simulink model "Vehicle_Model_Controller_Dec26"  (R2020b)
settings: Solver=VariableStepAuto  StartTime=0.0  StopTime=30  FixedStep=0.015  MaxStep=0.1  RelTol=1e-3
model workspace (MAT data in the model file):
  Kp = 10
  understeer_gradient = 0.05
undefined symbols (not defined in the file): BWL, BWR, FWL, FWR
libraries: fl_lib x32, nesl_utility x24, sdl_lib x8, pid_lib x1, vehdynlibsteering x1, autolibshared x1, autolibdatasheetbattery x1
(part 2 of 2)

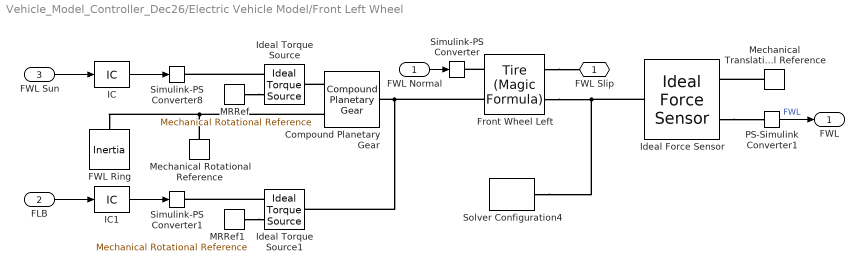
== system Vehicle_Model_Controller_Dec26/Electric Vehicle Model/Front Left Wheel ==
  FWL Normal : Inport
  FLB : Inport  Port=2
  FWL Sun : Inport  Port=3
  Compound Planetary Gear : sdl_lib/Gears/Compound Planetary Gear  rp_ratio=84/23  ps_ratio=37/24  friction_model=sdl.enum.gear_friction.none  mu_visc=[0, 0] N*m/(rad/s)  efficiency=[.96, .98]  temperature_TLU=[280, 300, 320] K  efficiency_sp_TLU=[.95, .9, .85]  efficiency_rp_TLU=[.95, .9, .85]  pwr_thr=[.001, .001] W  thermal_mass=50 J/K  T_init=300 K  model_inertia=simscape.enum.onoff.off  planet_inertia=0.001 kg*m^2
      settings: SourceProductBaseCode=LD  InternalSimscapePortConfiguration="{\"Bottom\":[],\"Left\":[{\"id\":\"C\",\"label\":\"C\",\"type\":\"foundation.mechanical.rotational.rotational\"}],\"Right\":[{\"id\":\"R\",\"label\":\"R\",\"type\":\"foundation.mechanical.rotational.rotational\"},{\"id\":\"S\",\"label\":\"S\",\"type\":\"foundation.mechanical.rotational.rotational\"}],\"Top\":[]}"
  FWL Ring : fl_lib/Mechanical/Rotational Elements/Inertia  inertia=0.1 kg*m^2  num_ports=foundation.enum.numPorts2.one  w_specify=off  w_priority=High  w=0 rad/s  w_nominal_specify=off  w_nominal_unit=rad/s  w_nominal_value=1  t_specify=off  t_priority=None  t=0 N*m  t_nominal_specify=off  t_nominal_unit=N*m  t_nominal_value=1
  Front Wheel Left : sdl_lib/Tires & Vehicles/Tire (Magic Formula)  parameterization=sdl.enum.magic_tire_model.constant  F_z1=3000 N  F_x1=3500 N  kappa1=10  B_m=10  C_m=1.9  D_m=1.5  E_m=0.97  fz0=4000 N  p_Cx=1.685  p_Dx=[1.21, -.037]  p_Ex=[.344, .095, -.02, 0]  p_Kx=[21.51, -.163, .245]  p_Hx=[-.002, .002]  p_Vx=[0, 0]  v_tr_thr=0.1 m/s  r_e=0.22 m  model_compliance=1  stiffness=2e5 N/m  damping=1000 N/(m/s)  model_inertia=1  inertia=0.03 kg*m^2  initial_velocity=0 rad/s  model_resistance=1  resistance_model=1  coeff=0.015  p_tire=82.74e3 Pa  alpha=-0.003  beta=0.97  coeff_a=84e-4  coeff_b=6.2e-4 s/m  coeff_c=1.6e-4 s^2/m^2  v_thr=0.01 m/s
  IC : InitialCondition  Value=0
  IC1 : InitialCondition  Value=0
  Ideal Force Sensor : fl_lib/Mechanical/Mechanical Sensors/Ideal Force Sensor
  Ideal Torque Source : fl_lib/Mechanical/Mechanical Sources/Ideal Torque Source
      settings: SourceProductName=Foundation Library
  Ideal Torque Source1 : fl_lib/Mechanical/Mechanical Sources/Ideal Torque Source
      settings: SourceProductName=Foundation Library
  MRRef : fl_lib/Mechanical/Rotational Elements/Mechanical Rotational Reference
      settings: SourceProductName=Foundation Library
  MRRef1 : fl_lib/Mechanical/Rotational Elements/Mechanical Rotational Reference
      settings: SourceProductName=Foundation Library
  Mechanical Rotational Reference : fl_lib/Mechanical/Rotational Elements/Mechanical Rotational Reference
  Mechanical Translational Reference : fl_lib/Mechanical/Translational Elements/Mechanical Translational Reference
  PS-Simulink Converter1 : nesl_utility/PS-Simulink Converter  PhysicalDomain=network_engine_domain  SubClassName=ps_output  LeftPortType=input  RightPortType=output  PseudoPeriodic=off  Frequencies=[]  Unit=inherit  AffineConversion=off
      settings: SourceProductBaseCode=PW,SS
  Simulink-PS Converter : nesl_utility/Simulink-PS Converter  PhysicalDomain=network_engine_domain  SubClassName=ps_input  LeftPortType=input  RightPortType=output  PseudoPeriodic=off  Frequencies=[]  NoiseDistribution=none  NoiseParameters=[]  Unit=N  AffineConversion=off  FilteringAndDerivatives=zero  SimscapeFilterOrder=1  InputFilterTimeConstant=0.001  UdotUserProvided=0
      settings: SourceProductBaseCode=PW,SS
  Simulink-PS Converter1 : nesl_utility/Simulink-PS Converter  PhysicalDomain=network_engine_domain  SubClassName=ps_input  LeftPortType=input  RightPortType=output  PseudoPeriodic=off  Frequencies=[]  NoiseDistribution=none  NoiseParameters=[]  Unit=N*m  AffineConversion=off  FilteringAndDerivatives=zero  SimscapeFilterOrder=1  InputFilterTimeConstant=0.001  UdotUserProvided=0
      settings: SourceProductBaseCode=PW,SS
  Simulink-PS Converter8 : nesl_utility/Simulink-PS Converter  PhysicalDomain=network_engine_domain  SubClassName=ps_input  LeftPortType=input  RightPortType=output  PseudoPeriodic=off  Frequencies=[]  NoiseDistribution=none  NoiseParameters=[]  Unit=N*m  AffineConversion=off  FilteringAndDerivatives=zero  SimscapeFilterOrder=1  InputFilterTimeConstant=0.001  UdotUserProvided=0
      settings: SourceProductBaseCode=PW,SS
  Solver Configuration4 : nesl_utility/Solver Configuration  PhysicalDomain=network_engine_domain  SubClassName=solver  LeftPortType=input  RightPortType=generic  Tones=[]  Harmonics=[]  SimulateNoise=off  Profile=off  UseLocalSampling=off  EnableSwitchedLinearOptims=on  FrequencyDomain=off  UseCCode=off  RelTol=0.001  AbsTol=1e-06  MinStep=1e-09  ToWorkspace=off  RevertToSquareIcSolve=off  NumHomotopyIterations=100  PhasorMode=off  PhasorModeNumHarmonics=1  DoDC=off  ResidualTolerance=1e-09  UseLocalSolver=off  LocalSolverChoice=NE_BACKWARD_EULER_ADVANCER  LocalSolverSampleTime=0.001  DoFixedCost=on  MaxNonlinIter=200  MaxModeIter=20  ComputeImpulses=off  ImpulseIterations=20  LinearAlgebra=auto  EquationFormulation=NE_TIME_EF  DelaysMemoryBudget=1024  AutomaticFiltering=on  FilteringTimeConstant=0.001  PartitionStorageMethod=AS_NEEDED  PartitionMemoryBudget=1024  PartitionMethod=ROBUST
      settings: SourceProductBaseCode=PW,SS
  FWL Slip : PMIOPort  Side=Left
  FWL : Outport
  wires:
  PS-Simulink Converter1/1 -> FWL/1  "FWL"
  FWL Normal/1 -> Simulink-PS Converter/1
  IC/1 -> Simulink-PS Converter8/1
  FWL Sun/1 -> IC/1
  IC1/1 -> Simulink-PS Converter1/1
  FLB/1 -> IC1/1
  connections:
  Front Wheel Left/RConn1 -- FWL Slip/RConn1
  Ideal Force Sensor/RConn2 -- PS-Simulink Converter1/LConn1
  Ideal Force Sensor/LConn1 -- Front Wheel Left/RConn2 -- Solver Configuration4/RConn1
  Front Wheel Left/LConn1 -- Simulink-PS Converter/RConn1
  Mechanical Translational Reference/LConn1 -- Ideal Force Sensor/RConn1
  Mechanical Rotational Reference/LConn1 -- FWL Ring/LConn1 -- Compound Planetary Gear/RConn1
  Ideal Torque Source/RConn1 -- Simulink-PS Converter8/RConn1
  Compound Planetary Gear/RConn2 -- Ideal Torque Source/LConn1
  MRRef/LConn1 -- Ideal Torque Source/RConn2
  Ideal Torque Source1/RConn1 -- Simulink-PS Converter1/RConn1
  MRRef1/LConn1 -- Ideal Torque Source1/RConn2
  Front Wheel Left/LConn2 -- Ideal Torque Source1/LConn1 -- Compound Planetary Gear/LConn1

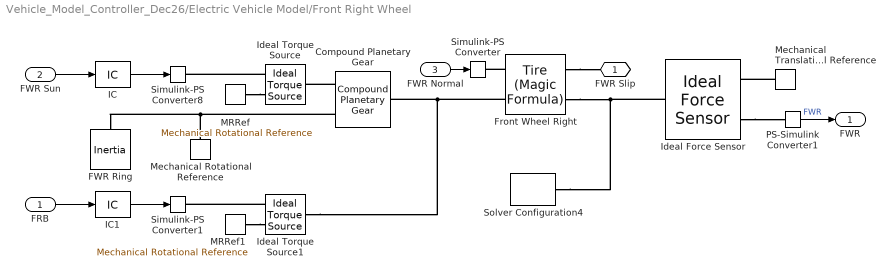
== system Vehicle_Model_Controller_Dec26/Electric Vehicle Model/Front Right Wheel ==
  FRB : Inport
  FWR Sun : Inport  Port=2
  FWR Normal : Inport  Port=3
  Compound Planetary Gear : sdl_lib/Gears/Compound Planetary Gear  rp_ratio=84/23  ps_ratio=37/24  friction_model=sdl.enum.gear_friction.none  mu_visc=[0, 0] N*m/(rad/s)  efficiency=[.96, .98]  temperature_TLU=[280, 300, 320] K  efficiency_sp_TLU=[.95, .9, .85]  efficiency_rp_TLU=[.95, .9, .85]  pwr_thr=[.001, .001] W  thermal_mass=50 J/K  T_init=300 K  model_inertia=simscape.enum.onoff.off  planet_inertia=0.001 kg*m^2
      settings: SourceProductBaseCode=LD  InternalSimscapePortConfiguration="{\"Bottom\":[],\"Left\":[{\"id\":\"C\",\"label\":\"C\",\"type\":\"foundation.mechanical.rotational.rotational\"}],\"Right\":[{\"id\":\"R\",\"label\":\"R\",\"type\":\"foundation.mechanical.rotational.rotational\"},{\"id\":\"S\",\"label\":\"S\",\"type\":\"foundation.mechanical.rotational.rotational\"}],\"Top\":[]}"
  FWR Ring : fl_lib/Mechanical/Rotational Elements/Inertia  inertia=0.1 kg*m^2  num_ports=foundation.enum.numPorts2.one  w_specify=off  w_priority=High  w=0 rad/s  w_nominal_specify=off  w_nominal_unit=rad/s  w_nominal_value=1  t_specify=off  t_priority=None  t=0 N*m  t_nominal_specify=off  t_nominal_unit=N*m  t_nominal_value=1
  Front Wheel Right : sdl_lib/Tires & Vehicles/Tire (Magic Formula)  parameterization=sdl.enum.magic_tire_model.constant  F_z1=3000 N  F_x1=3500 N  kappa1=10  B_m=10  C_m=1.9  D_m=1.5  E_m=0.97  fz0=4000 N  p_Cx=1.685  p_Dx=[1.21, -.037]  p_Ex=[.344, .095, -.02, 0]  p_Kx=[21.51, -.163, .245]  p_Hx=[-.002, .002]  p_Vx=[0, 0]  v_tr_thr=0.1 m/s  r_e=0.22 m  model_compliance=1  stiffness=2e5 N/m  damping=1000 N/(m/s)  model_inertia=1  inertia=0.03 kg*m^2  initial_velocity=0 rad/s  model_resistance=0  resistance_model=1  coeff=0.015  p_tire=82.74e3 Pa  alpha=-0.003  beta=0.97  coeff_a=84e-4  coeff_b=6.2e-4 s/m  coeff_c=1.6e-4 s^2/m^2  v_thr=0.001 m/s
  IC : InitialCondition  Value=0
  IC1 : InitialCondition  Value=0
  Ideal Force Sensor : fl_lib/Mechanical/Mechanical Sensors/Ideal Force Sensor
  Ideal Torque Source : fl_lib/Mechanical/Mechanical Sources/Ideal Torque Source
      settings: SourceProductName=Foundation Library
  Ideal Torque Source1 : fl_lib/Mechanical/Mechanical Sources/Ideal Torque Source
      settings: SourceProductName=Foundation Library
  MRRef : fl_lib/Mechanical/Rotational Elements/Mechanical Rotational Reference
      settings: SourceProductName=Foundation Library
  MRRef1 : fl_lib/Mechanical/Rotational Elements/Mechanical Rotational Reference
      settings: SourceProductName=Foundation Library
  Mechanical Rotational Reference : fl_lib/Mechanical/Rotational Elements/Mechanical Rotational Reference
  Mechanical Translational Reference : fl_lib/Mechanical/Translational Elements/Mechanical Translational Reference
  PS-Simulink Converter1 : nesl_utility/PS-Simulink Converter  PhysicalDomain=network_engine_domain  SubClassName=ps_output  LeftPortType=input  RightPortType=output  PseudoPeriodic=off  Frequencies=[]  Unit=inherit  AffineConversion=off
      settings: SourceProductBaseCode=PW,SS
  Simulink-PS Converter : nesl_utility/Simulink-PS Converter  PhysicalDomain=network_engine_domain  SubClassName=ps_input  LeftPortType=input  RightPortType=output  PseudoPeriodic=off  Frequencies=[]  NoiseDistribution=none  NoiseParameters=[]  Unit=N  AffineConversion=off  FilteringAndDerivatives=zero  SimscapeFilterOrder=1  InputFilterTimeConstant=0.001  UdotUserProvided=0
      settings: SourceProductBaseCode=PW,SS
  Simulink-PS Converter1 : nesl_utility/Simulink-PS Converter  PhysicalDomain=network_engine_domain  SubClassName=ps_input  LeftPortType=input  RightPortType=output  PseudoPeriodic=off  Frequencies=[]  NoiseDistribution=none  NoiseParameters=[]  Unit=N*m  AffineConversion=off  FilteringAndDerivatives=zero  SimscapeFilterOrder=1  InputFilterTimeConstant=0.001  UdotUserProvided=0
      settings: SourceProductBaseCode=PW,SS
  Simulink-PS Converter8 : nesl_utility/Simulink-PS Converter  PhysicalDomain=network_engine_domain  SubClassName=ps_input  LeftPortType=input  RightPortType=output  PseudoPeriodic=off  Frequencies=[]  NoiseDistribution=none  NoiseParameters=[]  Unit=N*m  AffineConversion=off  FilteringAndDerivatives=zero  SimscapeFilterOrder=1  InputFilterTimeConstant=0.001  UdotUserProvided=0
      settings: SourceProductBaseCode=PW,SS
  Solver Configuration4 : nesl_utility/Solver Configuration  PhysicalDomain=network_engine_domain  SubClassName=solver  LeftPortType=input  RightPortType=generic  Tones=[]  Harmonics=[]  SimulateNoise=off  Profile=off  UseLocalSampling=off  EnableSwitchedLinearOptims=on  FrequencyDomain=off  UseCCode=off  RelTol=0.001  AbsTol=1e-06  MinStep=1e-09  ToWorkspace=off  RevertToSquareIcSolve=off  NumHomotopyIterations=100  PhasorMode=off  PhasorModeNumHarmonics=1  DoDC=off  ResidualTolerance=1e-09  UseLocalSolver=off  LocalSolverChoice=NE_BACKWARD_EULER_ADVANCER  LocalSolverSampleTime=0.001  DoFixedCost=off  MaxNonlinIter=200  MaxModeIter=20  ComputeImpulses=off  ImpulseIterations=2  LinearAlgebra=auto  EquationFormulation=NE_TIME_EF  DelaysMemoryBudget=1024  AutomaticFiltering=on  FilteringTimeConstant=0.001  PartitionStorageMethod=AS_NEEDED  PartitionMemoryBudget=1024  PartitionMethod=ROBUST
      settings: SourceProductBaseCode=PW,SS
  FWR Slip : PMIOPort  Side=Right
  FWR : Outport
  wires:
  PS-Simulink Converter1/1 -> FWR/1  "FWR"
  FWR Normal/1 -> Simulink-PS Converter/1
  IC/1 -> Simulink-PS Converter8/1
  FWR Sun/1 -> IC/1
  IC1/1 -> Simulink-PS Converter1/1
  FRB/1 -> IC1/1
  connections:
  Front Wheel Right/RConn1 -- FWR Slip/RConn1
  Front Wheel Right/LConn1 -- Simulink-PS Converter/RConn1
  Ideal Force Sensor/RConn2 -- PS-Simulink Converter1/LConn1
  Ideal Force Sensor/LConn1 -- Front Wheel Right/RConn2 -- Solver Configuration4/RConn1
  Mechanical Translational Reference/LConn1 -- Ideal Force Sensor/RConn1
  MRRef/LConn1 -- Ideal Torque Source/RConn2
  Compound Planetary Gear/RConn2 -- Ideal Torque Source/LConn1
  Ideal Torque Source/RConn1 -- Simulink-PS Converter8/RConn1
  Front Wheel Right/LConn2 -- Ideal Torque Source1/LConn1 -- Compound Planetary Gear/LConn1
  Mechanical Rotational Reference/LConn1 -- FWR Ring/LConn1 -- Compound Planetary Gear/RConn1
  Ideal Torque Source1/RConn1 -- Simulink-PS Converter1/RConn1
  MRRef1/LConn1 -- Ideal Torque Source1/RConn2

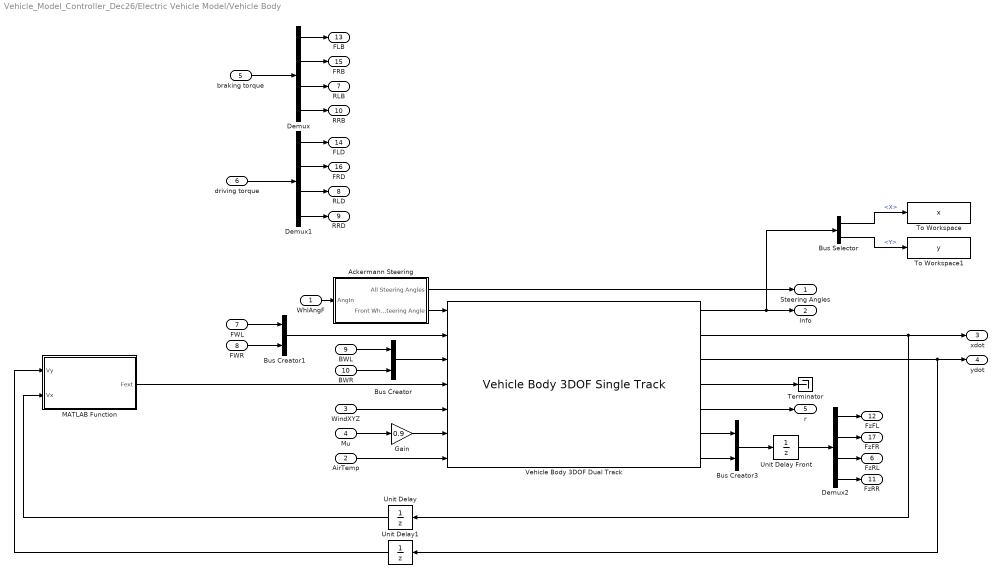
== system Vehicle_Model_Controller_Dec26/Electric Vehicle Model/Vehicle Body ==
  WhlAngF : Inport
  AirTemp : Inport  Port=2
  WindXYZ : Inport  Port=3
  Mu : Inport  Port=4
  braking torque : Inport  Port=5
  driving torque : Inport  Port=6
  FWL : Inport  Port=7
  FWR : Inport  Port=8
  BWL : Inport  Port=9
  BWR : Inport  Port=10
  Ackermann Steering : Subsystem
  Bus Creator : BusCreator  Inputs=BWL,BWR
  Bus Creator1 : BusCreator  Inputs=FWL,FWR
  Bus Creator3 : BusCreator  Inputs=2
  Bus Selector : BusSelector  OutputSignals=InertFrm.Cg.Disp.X,InertFrm.Cg.Disp.Y
  Demux : Demux
  Demux1 : Demux
  Demux2 : Demux
  Gain : Gain  Gain=0.9
  MATLAB Function : MATLAB Function  TreatAsAtomicUnit=on
  Terminator : Terminator
  To Workspace : ToWorkspace  VariableName=x  SaveFormat=Timeseries  SampleTime=-1
  To Workspace1 : ToWorkspace  VariableName=y  SaveFormat=Timeseries  SampleTime=-1
  Unit Delay : UnitDelay  SampleTime=-1  HasFrameUpgradeWarning=on
  Unit Delay Front : UnitDelay  InitialCondition=[547, 547, 547, 547]  SampleTime=-1  HasFrameUpgradeWarning=on
  Unit Delay1 : UnitDelay  SampleTime=-1  HasFrameUpgradeWarning=on
  Vehicle Body 3DOF Dual Track : autolibshared/Vehicle Body 3DOF Single Track  trackMode=Dual  inputMode=External longitudinal forces  frontSteerMode=on  rearSteerMode=off  windMode=on  muMode=on  extFMode=on  extMMode=off  htchFMode=off  htchMMode=off  extXo=off  extpsio=off  extxdoto=off  extro=off  extYo=off  extTamb=on  extydoto=off  aMode=2  NF=2  NR=2  m=308  a=0.7922471  b=0.7828529  h=0.295  dh=1  hh=0.2  X_o=0  xdot_o=0  CalphaMode=off  sigmaMode=on  d=0  hl=0  w=[1.29579,1.24204]  Cy_f=11e3  Cy_r=11e3  sigma_f=.1  sigma_r=.1  alpha_f_brk=[-.1 .1]  Cy_f_data=[-9e3 9e3]  alpha_r_brk=[-.1 .1]  Cy_r_data=[-9e3 9e3]  Y_o=0  ydot_o=0  Izz=4000  psi_o=0  r_o=0  Af=1.0221  Cd=1.149  Cl=0  Cpm=.000001  beta_w=[0:0.01:0.3]  Cs=[0:0.03:0.9]  Cym=[0:0.01:0.3]  Pabs=101325  Tair=273  g=9.81  mu=1  xdot_tol=.1  Fznom=15000  Fxtire_sat=7e4  Fytire_sat=7e4  longOff=0  latOff=0  vertOff=0  wrapAng=off
      settings: SourceProductBaseCode=PW,DR,MT,UV,VE
  Steering Angles : Outport
  Info : Outport  Port=2
  xdot : Outport  Port=3
  ydot : Outport  Port=4
  r : Outport  Port=5
  FzRL : Outport  Port=6
  RLB : Outport  Port=7
  RLD : Outport  Port=8
  RRD : Outport  Port=9
  RRB : Outport  Port=10
  FzRR : Outport  Port=11
  FzFL : Outport  Port=12
  FLB : Outport  Port=13
  FLD : Outport  Port=14
  FRB : Outport  Port=15
  FRD : Outport  Port=16
  FzFR : Outport  Port=17
  wires:
  Vehicle Body 3DOF Dual Track/3 -> Unit Delay1/1, ydot/1
  Bus Creator1/1 -> Vehicle Body 3DOF Dual Track/2
  Vehicle Body 3DOF Dual Track/1 -> Info/1, Bus Selector/1
  AirTemp/1 -> Vehicle Body 3DOF Dual Track/7
  Vehicle Body 3DOF Dual Track/4 -> Terminator/1
  Vehicle Body 3DOF Dual Track/5 -> r/1
  Bus Creator/1 -> Vehicle Body 3DOF Dual Track/3
  Ackermann Steering/2(Front Wheels Steering Angle) -> Vehicle Body 3DOF Dual Track/1
  WindXYZ/1 -> Vehicle Body 3DOF Dual Track/5
  Demux2/1 -> FzFL/1
  Demux2/2 -> FzFR/1
  FWL/1 -> Bus Creator1/1
  FWR/1 -> Bus Creator1/2
  Demux2/3 -> FzRL/1
  Demux2/4 -> FzRR/1
  BWL/1 -> Bus Creator/1
  BWR/1 -> Bus Creator/2
  Gain/1 -> Vehicle Body 3DOF Dual Track/6
  Mu/1 -> Gain/1
  Ackermann Steering/1(All Steering Angles) -> Steering Angles/1
  WhlAngF/1 -> Ackermann Steering/1(AngIn)
  Bus Selector/1 -> To Workspace/1  "<X>"
  Bus Selector/2 -> To Workspace1/1  "<Y>"
  Vehicle Body 3DOF Dual Track/7 -> Bus Creator3/2
  Vehicle Body 3DOF Dual Track/6 -> Bus Creator3/1
  Bus Creator3/1 -> Unit Delay Front/1
  Unit Delay Front/1 -> Demux2/1
  MATLAB Function/1(Fext) -> Vehicle Body 3DOF Dual Track/4
  Unit Delay/1 -> MATLAB Function/2(Vx)
  Unit Delay1/1 -> MATLAB Function/1(Vy)
  Vehicle Body 3DOF Dual Track/2 -> xdot/1, Unit Delay/1
  driving torque/1 -> Demux1/1
  braking torque/1 -> Demux/1
  Demux/1 -> FLB/1
  Demux/2 -> FRB/1
  Demux/3 -> RLB/1
  Demux/4 -> RRB/1
  Demux1/1 -> FLD/1
  Demux1/2 -> FRD/1
  Demux1/3 -> RLD/1
  Demux1/4 -> RRD/1

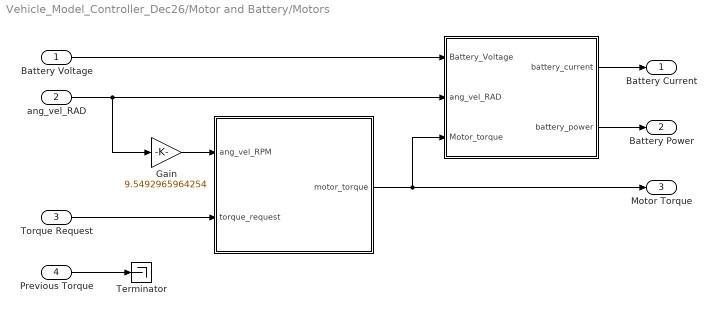
== system Vehicle_Model_Controller_Dec26/Motor and Battery/Motors ==
  Battery Voltage : Inport
  ang_vel_RAD : Inport  Port=2
  Torque Request : Inport  Port=3
  Previous Torque : Inport  Port=4
  " " : MATLAB Function  TreatAsAtomicUnit=on
  "  " : MATLAB Function  TreatAsAtomicUnit=on
  Gain : Gain  Gain=9.5492965964254
  Terminator : Terminator
  Battery Current : Outport
  Battery Power : Outport  Port=2
  Motor Torque : Outport  Port=3
  wires:
  Torque Request/1 -> " "/2(torque_request)
  Battery Voltage/1 -> "  "/1(Battery_Voltage)
  ang_vel_RAD/1 -> Gain/1, "  "/2(ang_vel_RAD)
  "  "/1(battery_current) -> Battery Current/1
  " "/1(motor_torque) -> Motor Torque/1, "  "/3(Motor_torque)
  "  "/2(battery_power) -> Battery Power/1
  Gain/1 -> " "/1(ang_vel_RPM)
  Previous Torque/1 -> Terminator/1

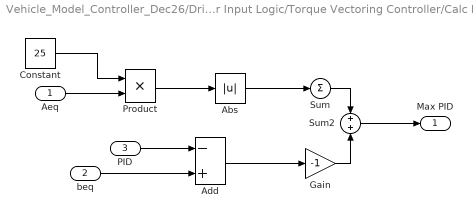
== system Vehicle_Model_Controller_Dec26/Driver Input Logic/Torque Vectoring Controller/Calc Max PID ==
  Aeq : Inport
  beq : Inport  Port=2
  PID : Inport  Port=3
  Abs : Abs
  Add : Sum  Inputs=-+
  Constant : Constant  Value=25
  Gain : Gain  Gain=-1
  Product : Product
  Sum : Sum  Inputs=1
  Sum2 : Sum
  Max PID : Outport
  wires:
  Add/1 -> Gain/1
  Product/1 -> Abs/1
  PID/1 -> Add/1
  Abs/1 -> Sum/1
  Sum2/1 -> Max PID/1
  Gain/1 -> Sum2/2
  Sum/1 -> Sum2/1
  Aeq/1 -> Product/2
  Constant/1 -> Product/1
  beq/1 -> Add/2

== system Vehicle_Model_Controller_Dec26/Driver Input Logic/Torque Vectoring Controller/Calc Power Consumption ==
  Required Torque : Inport
  Motor Shaft Velocity : Inport  Port=2
  Product : Product
  Sum : Sum  Inputs=|+
  Transpose : Math  Operator=transpose  SaturateOnIntegerOverflow=on
  Power : Outport
  wires:
  Product/1 -> Sum/1
  Motor Shaft Velocity/1 -> Transpose/1
  Transpose/1 -> Product/2
  Required Torque/1 -> Product/1
  Sum/1 -> Power/1

== system Vehicle_Model_Controller_Dec26/Electric Vehicle Model/Vehicle Body/Ackermann Steering ==
  AngIn : Inport
  Bus Creator : BusCreator  Inputs=2
  Deg to Rad : Gain  Gain=pi/180
  Kinematic Steering : vehdynlibsteering/Kinematic Steering  StrgType=Ackerman  StrgRatioType=Constant  Loc=Front  NrmlFctr=1  TrckWdth=1.29579  WhlBase=1.5751  Db=0  StrgRng=1.25*pi  StrgAngBpts="[-6.2832   -5.0265   -3.7699   -2.5133   -1.2566         0    1.2566    2.5133    3.7699    5.0265    6.2832]"  StrgRatioTbl=|  StrgRatio=1  StrgArmLngth=0.1  RckCsLngth=0.5  TieRodLngth=0.248  D=0.2  PnnRadius=0.0057  PnnRadiusTbl="[0.0055    0.0055    0.0056    0.0057    0.0058    0.0057    0.0057    0.0057    0.0056    0.0055    0.0055]"  RodLngth=0.1  ParaArmLngth=0.9  aMode=2
      | [13.5000   13.3750   13.2500   13.1250   13.0000   13.0000   13.0000   13.1250   13.2500   13.3750   13.5000
      | ]
  Mux3 : Mux  Inputs=2
  Terminator : Terminator
  All Steering Angles : Outport
  Front Wheels Steering Angle : Outport  Port=2
  wires:
  Kinematic Steering/2 -> Mux3/1
  Kinematic Steering/3 -> Mux3/2
  Kinematic Steering/1 -> Terminator/1
  Mux3/1 -> Front Wheels Steering Angle/1, Bus Creator/1  "ackermann angles"
  Bus Creator/1 -> All Steering Angles/1
  Deg to Rad/1 -> Kinematic Steering/1, Bus Creator/2  "steering_angle"
  AngIn/1 -> Deg to Rad/1  "steering_angle"

== matlab function Vehicle_Model_Controller_Dec26/Driver Input Logic/Torque Vectoring Controller/Layer 2 ==
  data: prev_torque output; driver_input output; power_limit_battery output; Fy_wheel output; omega_m output size=[1 4]; x output; y output; T2F output; slip_limit output; torque_limit_motor output; tau_limit_upper output; tau_limit_lower output; prev_torque input; driver_input input; power_limits_battery input; center_steer_angle input; acker_steer_angles input; Fx input; Fy input; vel input; T2F input; F_max input; T_brake input; yaw input; yaw_ref input; yaw_err output; motor_limit_power data_store_memory; motor_efficiency data_store_memory; s data_store_memory; J_z data_store_memory; gr data_store_memory; r data_store_memory; tau data_store_memory; motor_limit_torque data_store_memory; f data_store_memory; l data_store_memory; disk_diameter data_store_memory
function [prev_torque, driver_input, power_limit_battery, Fy_wheel, omega_m, x, y, T2F, slip_limit, torque_limit_motor, tau_limit_upper, tau_limit_lower, yaw_err] = Layer_2(prev_torque, driver_input, power_limits_battery, center_steer_angle, acker_steer_angles, Fx, Fy, vel, T2F, F_max, T_brake, yaw, yaw_ref)
%% Layer 2 Computation
% Developer(s):    David Farell
%                  Demetrius Gulewicz
%                  Elliot Stockwell
%                  Tao Sun
%
% Developed for: Purdue Electric Racing
% Date:          12/25/2021
%
% Description: This function primarily computes the maximum and minimum
%              torque that can be requested, based on slip, power, and 
%              transient constraints. Also computes yaw error.
%
%
%% Pass Through Signals
% prev_torque - Torque requested to motor in previous time step [Nm][4x1]
% driver_input - Proportion Of Total Absolute Power To Use [Unitless][1x1]
% T2F - Convert Torque At The Motor Shaft to Force At The Tire [1/m][1x4]
%
%
%% Input Only
% power_limits_battery - Max & Min Total Battery Power Output [W][1x2]
% center_steer_angle - Steering Column Angle From Neutral [rad][1x1]
% acker_steer_angles - Angle Tires Are Turned From Neutral [rad][1x2]
% Fx - Tires Forces x Direction, Vehicle Fixed Coordinates [N][1x4]
% Fy - Tires Forces y Direction, Vehicle Fixed Coordinates [N][1x4]
% vel - Velocity Of Tires, Vehicle Fixed Coordinates [m/s][1x6]
% yaw - Yaw Rate z Direction, Vehicle Fixed Coordinates  [rad/s][1x1]
% F_max - Max Allowed Force On Each Tire-Ground Contact Plane [N][1x4]
% T_brake - Mechanical Brake Torque On Each Tire [Nm][1x4]
% yaw_ref - The Desired & Max Allowed Yaw Rate [rad/s][1x2]
%
%
%% Output Only:
% power_limit_battery - Max OR Min Total Battery Power Output [W][1x1]
% Fy_wheel - Tires forces y direction, Tire fixed coordinates [N][1x4]
% omega_m - Motor Shaft Angular Velocity [rad/s][1x4]
% x - Equivalent Distances That Fx Acts From CoG [m][1x4]
% y - Equivalent Distances That Fy Acts From CoG [m][1x4] 
% slip_limit - Max Torque Before Tire Slips [Nm][1x4]
% torque_limit_motor - Max Torque Motor Can Output [Nm][1x4]
% tau_limit_upper - Max Torque Motor Is Allowed To Change To [Nm][1x4]
% tau_limit_lower - Min Torque Motor Is Allowed To Change To [Nm][1x4]
% yaw_err - Error Between Target & Actual Yaw Rate [rad/s][1x1]
%
%
%% Constants
global s; % Half track width [m][1x2]
global l; % Wheelbase [m][1x2]
global motor_limit_power; % Absolute Power Limit For Each Motor [W][1x4]
global motor_efficiency; % Motor Efficiency [Unitless][1x4]
global tau; % Motor Response Time Constant [s][1x1]
global f; % Controller Frequency [Hz][1x1]
global gr; % Gear Ratios [Unitless][1x4]
global r; % Tire Radius [m][1x1]
global motor_limit_torque; % Min & Max Torque Request From Motor [Nm][1x2]


%% Calculations
% Calculate the Yaw Error, Apply Sign Convention
if yaw_ref(1) == 0 && yaw(1) == 0
    yaw_err = 0;
elseif center_steer_angle >= 0
    yaw_err = min(abs(yaw_ref)) - yaw;
else
    yaw_err = (min(abs(yaw_ref)) * -1) - yaw;
end

% Motor Shaft Speed, RAD/S
omega_fl = (vel(1) * cos(acker_steer_angles(1))) + (vel(2) * sin(acker_steer_angles(1)));
omega_fr = (vel(3) * cos(acker_steer_angles(2))) + (vel(4) * sin(acker_steer_angles(2)));
omega_rl = vel(5);
omega_rr = vel(6);
omega_m = [omega_fl, omega_fr, omega_rl, omega_rr] .* (gr ./ r);

% Calculate K_1 Vehicle Constants
x_1 = (s(1) * cos(acker_steer_angles(1))) + (l(1) * sin(acker_steer_angles(1)));
x_2 = (-1 * s(1) * cos(acker_steer_angles(2))) + (l(1) * sin(acker_steer_angles(2)));
x_3 = s(2);
x_4 = -s(2);
x = [x_1, x_2, x_3, x_4]; 

% Get Lateral Forces Acting On Vehicle In Tire Coordinate System
F_y_ij_fl = (-sin(acker_steer_angles(1)) * Fx(1)) + (cos(acker_steer_angles(1)) * Fy(1));
F_y_ij_fr = (-sin(acker_steer_angles(2)) * Fx(2)) + (cos(acker_steer_angles(2)) * Fy(2));
F_y_ij_rl = Fy(3);
F_y_ij_rr = Fy(4);
Fy_wheel = [F_y_ij_fl, F_y_ij_fr, F_y_ij_rl, F_y_ij_rr];

% Calculate K_2 Vehicle Constants
y_1 = (-1 * s(1) * sin(acker_steer_angles(1))) + (l(1) * cos(acker_steer_angles(1)));    
y_2 = (s(1) * sin(acker_steer_angles(2))) + (l(1) * cos(acker_steer_angles(2)));
y_3 = -l(2);
y_4 = -l(2);
y = [y_1, y_2, y_3, y_4]; 

% Longitudinal Force Limits On Individual Tires Due To Friction
Fx_max2 = (F_max.^2)-(Fy_wheel.^2);

% Control For Negative Output
for i = 1:4
    if Fx_max2(i) < 0
        Fx_max2(i) = 0;
    end
end

% Calculate Torque Limit Due to Power and Slip
Fx_max = sqrt(Fx_max2)-(T_brake./r);
slip_limit = Fx_max ./ T2F; 
torque_limit_motor = (motor_limit_power .* motor_efficiency) ./ omega_m;


% Erase power limit solution above torque limit, for better data
% visualization
for i = 1:4
    if torque_limit_motor(i) > 25 
        torque_limit_motor(i) = 25;
    elseif torque_limit_motor(i) < -25
        torque_limit_motor(i) = -0.01; 
    end
end 

% Calculate Constants for getting limit on motor output torque due to
% motor response time
% Note: e_term, c_lower, c_upper are based on tunable parameters, during
% runtime, they are constant
e_term = exp(-1 / (tau * f));
c_lower = (1 - e_term) .* motor_limit_torque(1);
c_upper = (1 - e_term) .* motor_limit_torque(2);
c_constant = (prev_torque .* e_term)';

% Max and Min Torque Limits due to motor response time
tau_limit_upper = max([c_upper + c_constant; c_constant + .01]);
tau_limit_lower = min([c_lower + c_constant; c_constant - .01]);

% If driver is not pressing acceleration pedal, no positive torque is allowed
if driver_input <= 0
   tau_limit_upper = [0, 0, 0, 0];
   power_limit_battery = power_limits_battery(2);  
else
    power_limit_battery = power_limits_battery(1);
end

end

== matlab function Vehicle_Model_Controller_Dec26/Electric Vehicle Model/Vehicle Body/MATLAB Function ==
  data: Vy input; Vx input; Fext output
function Fext = get_downforce(Vy, Vx)
%% Constants
rho = 1.225; % Air density [Kg/m^3]
cl = 2.11014; % Lift coefficient [unitless]
A = 1.0221; % Frontal Area [m^2]


%% Computation
% Compute CoG Velocity
Vcog = Vx^2 + Vy^2;

% Compute DownForce
Fz = 0.5 * rho * Vcog * cl * A;
Fext = [0, 0, Fz];

== matlab function Vehicle_Model_Controller_Dec26/Motor and Battery/Motors/  ==
  data: ang_vel_RPM input; motor_torque output size=[1 4]; torque_request input
function motor_torque = get_torque(ang_vel_RPM, torque_request)
%% Actual Torque Output
% Developers:    Demetrius Gulewicz

% Developed for: Purdue Electric Racing
% Date:          09/18/2021
%
% Definitions:
% ang_vel:   Angular velocity of each wheel on the wheel fixed y axis [RPM]
% torque_request: Requested torque from the LP model                  [Nm]

%% Constants
% quadratic constants that connect current and max RPM of motors
a_v = 0.2667;
b_v = -66.353;
c_v = 10452 - ang_vel_RPM;

% quadratic constants that connnect current and max torque of motors
a_t = -0.0987;
b_t = 45.799;
c_t = -129.65;

% maximum possible current at the current RPM
max_current = [0, 0, 0, 0];


%% Calculate Maximum Torque Possible
% calculate the maximum current possible at the current RPM
for i = [1:4]
   if ang_vel_RPM(i) < 7000
       max_current(i) = 70;
   else
       max_current(i) = (-b_v - sqrt(b_v^2 - (4*a_v.*c_v(i)))) .* (1/(2*a_v));
   end
end

% calculate the meximum torque at the max current
max_torque = (a_t .* (max_current.^2)) + (b_t .* max_current) + c_t;
for i = [1:4]
   if max_torque(i) < 0
      max_torque(i) = 0;
   end
end

motor_torque_matrix = [max_torque; torque_request'];
motor_torque = min(motor_torque_matrix);

== matlab function Vehicle_Model_Controller_Dec26/Driver Input Logic/Torque Vectoring Controller/LP_Calc  ==
  data: prev_torque input; driver_input input; power_limit_battery input; Fy_wheel input; omega_m input; x input; y input; T2F input; slip_limit input; power_limit input; tau_limit_upper input; tau_limit_lower input; Tx output size=[4 1]; omega_m output; lb output double; PID input; ub output double; Aeq output double; beq output double; A output; b output; M_max output; J_z data_store_memory; motor_efficiency data_store_memory; motor_limit_torque data_store_memory; min_speed_regen data_store_memory
function [Tx, omega_m, lb, ub, Aeq, beq, A, b, M_max] = LP_calc(prev_torque, driver_input, power_limit_battery, Fy_wheel, omega_m, x, y, T2F, slip_limit, power_limit, tau_limit_upper, tau_limit_lower, PID)
%% LP_calc Computation
% Developer(s):    David Farell
%                  Demetrius Gulewicz
%                  Elliot Stockwell
%                  Tao Sun
%
% Developed for: Purdue Electric Racing
% Date:          12/25/2021
%
% Description: This function primarily computes the desired torque
%              distribution after constructing an optimization statement.
%
%
%% Pass Through Signals
% omega_m - Motor Shaft Angular Velocity [rad/s][1x4]
%
%
%% Input Only:
% prev_torque - Torque Requested To Motor In Previous Time Step [Nm][4x1]
% driver_input - Proportion of total power to use [Unitless][1x1]
% T2F - Convert Torque At The Motor Shaft to Force At The Tire [1/m][1x4]
% power_limit_battery - Max & Min Total Battery Power Output [W][1x2]
% Fy_wheel - Tires Forces y Direction, Tire fixed coordinates [N][1x4]
% x - Equivalent Distances That Fx Acts From CoG [m][1x4]
% y - Equivalent Distances That Fy Acts From CoG [m][1x4]
% slip_limit - Max Torque Before Tire Slips [Nm][1x4]
% torque_limit_motor - Max Torque Motor Can Output [Nm][1x4]
% tau_limit_upper - Max Torque Motor Is Allowed To Change To [Nm][1x4]
% tau_limit_lower - Min Torque Motor Is Allowed To Change To [Nm][1x4]
% PID - Desired Yaw Acceleration [rad/s^2][1x1]
%
%
%% Output Only:
% Tx - Torque Request To Motors [Nm][4x1]
% lb - Min Torque Request [Nm][1x4]
% ub - Max Torque Request [Nm][1x4]
% Aeq - Moment About CoG, Optimization Variable [rad/s^2][1x1]
% beq - Moment About CoG, Yaw Acceleration & Other Foces [rad/s^2][1x1]
% A - Power Consumed, Optimization Variable [W][1x1]
% b - Power Consumed, Driver Input [W][1x1]
% M_max - Max & Min Yaw Acceleration Achievable With lb & ub [rad/s^2][1x2]
%
%
%% Constants
global J_z; % Polar Moment Of Inertia [kg m^2][1x1]
global motor_efficiency; % Motor efficiency [Unitless][1x4]
global motor_limit_torque; % Minimum & Max Torque Request From Motor [Nm][1x2]
global min_speed_regen; % Min Motor Shaft Speed For Regen Braking [rad/s][1x1]


%% Calculation
% Calculate Boundary Conditions, The Max and Min Allowable Torque
ub = [0, 0, 0, 0];
lb = [0, 0, 0, 0];

for i = 1:4
    ub(i) = min([slip_limit(i), power_limit(i), motor_limit_torque(2), tau_limit_upper(i)]);
    lb(i) = max([-slip_limit(i), -power_limit(i), motor_limit_torque(1), tau_limit_lower(i)]);
end

% Enforce No Backwards Rotation Of Tires
for i = 1:4
   if omega_m(i) < min_speed_regen && lb(i) < -0.1
       lb(i) = -0.001;
   end
end

% Max & Min Forces on the Tires
ub_f = ub .* T2F;
lb_f = lb .* T2F;

% Find Max & Min For PID, The Yaw Acceleration Of The Car
M_max=zeros(1,2);
M_max(1) = (x(1)*ub_f(1)+x(3)*ub_f(3)+x(2)*lb_f(2)+x(4)*lb_f(4)+sum(y.*Fy_wheel))/J_z;
M_max(2) = (x(2)*ub_f(2)+x(4)*ub_f(4)+x(1)*lb_f(1)+x(3)*lb_f(3)+sum(y.*Fy_wheel))/J_z;

% Limit PID To Be No Larger Than Possible Due To Torque Constraints
if PID >= M_max(1)
    PID = M_max(1);
elseif PID <= M_max(2)
    PID = M_max(2);
end

% Calculate Yaw Constraint
Aeq = ((1 ./ J_z) .* x) .* T2F;
beq = PID-sum(((1 / J_z) * y) .* Fy_wheel);

% Calculate Power Constraint
if driver_input >=0
    A = omega_m ./ motor_efficiency;
else 
    A = -omega_m ./ motor_efficiency;
end
b = driver_input*power_limit_battery;


%% Optimization
% Set Optimization Parameters
options = optimoptions('fmincon','Algorithm','sqp');

% Determine correct objective function maximize the forces acting on the car
if driver_input >= 0
    objfun = @(q) -sum(q .* T2F);
    Tx = fmincon(objfun,prev_torque',A,b,Aeq,beq,lb,ub,[],options)';
else 
    objfun = @(q) sum(q .* T2F);    
    Tx = fmincon(objfun,prev_torque',A,b,Aeq,beq,lb,ub,[],options)';
end 

end

== matlab function Vehicle_Model_Controller_Dec26/Motor and Battery/Motors/   ==
  data: Battery_Voltage input; ang_vel_RAD input; battery_current output; Motor_torque input; battery_power output
function [battery_current, battery_power]= get_batt_curr(Battery_Voltage, ang_vel_RAD, Motor_torque)
%% Current Draw
% Developers:    Demetrius Gulewicz

% Developed for: Purdue Electric Racing
% Date:          09/18/2021
%
% Definitions:
% ang_vel_RAD:   Angular velocity of each wheel on the wheel fixed y axis [RAD]
% Motor_torque:  Torque the motor actually outputs                 [Ncm]
% Battery_Voltage: The voltage of the battery                      [V]

%% Definitions
a = 0.0411;
b = 2.7976;
c = 45.978;

t = Motor_torque;
w = ang_vel_RAD;
v = Battery_Voltage;

e = 85;

%% Calculate Current Draw
%x0 = [20, 20, 20, 20];
%options = optimoptions('fsolve','Algorithm','Levenberg-Marquardt');
%F = @(x) ([(a * x(1)^3) + (b * x(1)^2) + (c * x(1)), ] .* v) - (t .* w);
%battery_current = sum(fsolve(F,x0,options));

battery_current = sum((t .* w') ./ (e .* v));
battery_power = battery_current * Battery_Voltage;
end

== matlab function Vehicle_Model_Controller_Dec26/Driver Input Logic/Torque Vectoring Controller/Layer 1 ==
  data: driver_input output; power_limits_battery output; center_steer_angle output; acker_steer_angles output; Fx output; Fy output; vel output; T2F output; F_max output; T_brake output size=[1 4]; yaw output; yaw_ref output; driver_input input; power_limits_battery input; center_steer_angle input; acker_steer_angles input; Fx input; Fy input; Fz input; vel input; Vx input; Vy input; yaw input; K_u data_store_memory; gr data_store_memory; gearbox_efficiency data_store_memory; tau data_store_memory; f data_store_memory; c_factor data_store_memory; J_z data_store_memory; l data_store_memory; s data_store_memory; r data_store_memory; g data_store_memory; tire_mu data_store_memory; brakeforce_max data_store_memory; brakepad_mu data_store_memory; disk_diameter data_store_memory; mech_brake data_store_memory
function [driver_input, power_limits_battery, center_steer_angle, acker_steer_angles, Fx, Fy, vel, T2F, F_max, T_brake, yaw, yaw_ref] = Layer_1(driver_input, power_limits_battery, center_steer_angle, acker_steer_angles, Fx, Fy, Fz, vel, Vx, Vy, yaw)
%% Layer 1 Computation
% Developer(s):    David Farell
%                  Demetrius Gulewicz
%                  Elliot Stockwell
%                  Tao Sun
%
% Developed for: Purdue Electric Racing
% Date:          12/25/2021
%
% Description: This function primarily computes the reference yaw rate, 
%              and the brake forces & distribution.
%
%
%% Pass Through Signals
% driver_input - Proportion Of Total Absolute Power To Use [Unitless][1x1]
% power_limits_battery - Max & Min Total Battery Power Output [W][1x2]
% center_steer_angle - Steering Column Angle From Neutral [rad][1x1]
% acker_steer_angles - Angle Tires Are Turned From Neutral [rad][1x2]
% Fx - Tires Forces x Direction, Vehicle Fixed Coordinates [N][1x4]
% Fy - Tires Forces y Direction, Vehicle Fixed Coordinates [N][1x4]
% vel - Velocity Of Tires, Vehicle Fixed Coordinates [m/s][1x6]
% yaw - Yaw Rate z Direction, Vehicle Fixed Coordinates  [rad/s][1x1]
%
%
%% Input Only:
% Fz - Tires Forces z Direction, Vehicle Fixed Coordinates [N][1x4]
% Vx - Center Of Gravity x Velocity, Vehicle Fixed Coordinates [m/s][1x1]
% Vy - Center Of Gravity y Velocity, Vehicle Fixed Coordinates [m/s][1x1]
%
%
%% Output Only: 
% T2F - Convert Torque At The Motor Shaft to Force At The Tire [1/m][1x4]
% F_max - Max Allowed Force On Each Tire-Ground Contact Plane [N][1x4]
% T_brake - Mechanical Brake Torque On Each Tire [Nm][1x4]
% yaw_ref - The Desired & Max Allowed Yaw Rate [rad/s][1x2]
%
%
%% Constants
global g; % Acceleration Due To Gravity [m/s^2][1x1]
global tire_mu; % Maximum Friction Coefficient [Unitless][1x4]
global gr; % Gear ratios [Unitless][1x4]
global gearbox_efficiency; % Gearbox Power Transmission Efficiency [Unitless][1x4]
global r; % Tire Radius [m][1x1]
global l; % Wheelbase [m][1x2]
global K_u; % Understeer Gradient [rad/m/s^2][1x1]
global c_factor; % Max Yaw Equation Contributing Factor [Unitless][1x1]
global brakeforce_max; % Max Force Brakes Can Exert On Each Tire Axle [N][1x4]
global brakepad_mu; % Brakepad Friction Coefficient[Unitless][1x1]
global mech_brake; % Value Of driver_input Where Mechanical Braking Begins [Unitless][1x1]
global disk_diameter; % Diameter of brake disk [m][1x1]


%% Calculation
% Max Allowed Force On Each Tire-Ground Contact Plane
F_max = abs(tire_mu.*Fz)';

% Convert Torque At The Motor Shaft to Force At The Wheel
% During Runtime, T2F Is Constant
T2F = (gr .* gearbox_efficiency) ./ r;

% Yaw Calculations
v_cog = sqrt(Vx^2 + Vy^2);
yaw_des = (v_cog * abs(center_steer_angle)) / ((l(1) + l(2)) + (K_u * v_cog ^ 2));
yaw_max = (c_factor * max(tire_mu) * g) / (v_cog);

% Control For Large Max Yaw, For Better Viewing
if yaw_max > 1
    yaw_max = 1;
end

yaw_ref = [yaw_des, yaw_max];

% Compute brake force and distribution
% for small brakes (input >= mech_brake), only regen braking
% for large brakes (input <= mech_brake), regen & mechanical braking
% note: actual force may not be proportional to the input
T_brake = [0,0,0,0];

if driver_input <= mech_brake   
    brakeforce_ratio = [1, 1, 1, 1] .* -(driver_input - mech_brake) / (1 + mech_brake);
    T_brake = -1.*brakeforce_ratio.*brakeforce_max.*brakepad_mu.*sqrt(abs(Vx)).*disk_diameter;
    driver_input = -1;
end

if Vx < 0
    T_brake = -T_brake;
end

if driver_input <= 0 && driver_input >= mech_brake
    driver_input = -driver_input / mech_brake;  % in scale of [-1,0]
end

end
